simulink model "project3"  (R2017a)
settings: Solver=ode45  StartTime=0.0  StopTime=1000  FixedStep=.1  RelTol=1e-3
libraries: simulink x6
settings Model: Creator=pizzaslayer  LastModifiedBy=pizzaslayer

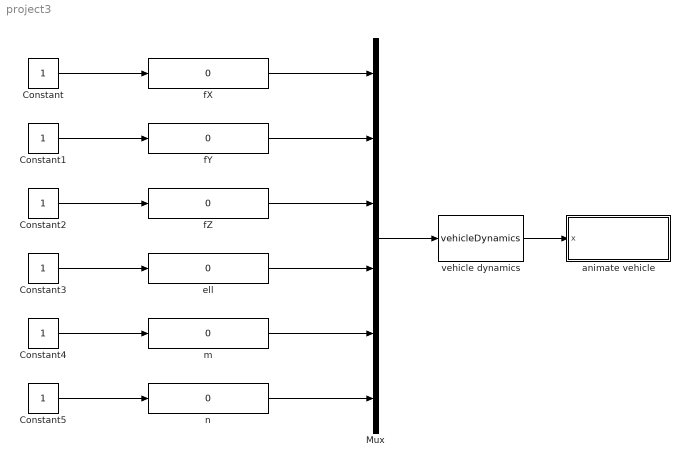
== system project3 ==
  Constant{,1..5} (6 alike) : Constant
  Mux : Mux  Inputs=6
  "animate vehicle " : Subsystem
  ell : simulink/Math Operations/Slider Gain  gain=0  low=-10  high=10
  fX : simulink/Math Operations/Slider Gain  gain=0  low=-10  high=10
  fY : simulink/Math Operations/Slider Gain  gain=0  low=-10  high=10
  fZ : simulink/Math Operations/Slider Gain  gain=0  low=-10  high=10
  m : simulink/Math Operations/Slider Gain  gain=0  low=-10  high=10
  n : simulink/Math Operations/Slider Gain  gain=0  low=-10  high=10
  vehicle dynamics : S-Function  FunctionName=vehicleDynamics  Parameters=P  SFunctionDeploymentMode=off  EnableBusSupport=off
  wires:
  fX/1 -> Mux/1
  Constant/1 -> fX/1
  Constant1/1 -> fY/1
  fY/1 -> Mux/2
  fZ/1 -> Mux/3
  Constant2/1 -> fZ/1
  ell/1 -> Mux/4
  Constant3/1 -> ell/1
  Constant4/1 -> m/1
  Constant5/1 -> n/1
  m/1 -> Mux/5
  n/1 -> Mux/6
  Mux/1 -> vehicle dynamics/1
  vehicle dynamics/1 -> "animate vehicle "/1(x)

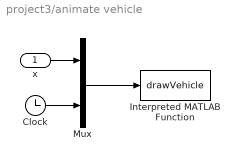
== system project3/animate vehicle  ==
  x : Inport
  Clock : Clock
  Interpreted MATLAB Function : MATLABFcn  MATLABFcn=drawVehicle  OutputDimensions=0
  Mux : Mux  Inputs=2
  wires:
  x/1 -> Mux/1
  Clock/1 -> Mux/2
  Mux/1 -> Interpreted MATLAB Function/1
